simulink model "Copy_of_MMC_test_v3"  (R2020b)
settings: Solver=ode1  StartTime=0.0  StopTime=4  FixedStep=10e-6  RelTol=1e-3
undefined symbols (not defined in the file): DiscIntNeverNeededParam, GRD00_Lg, GRD00_Rg, VSC01_id0
libraries: MMC x12, spsSeriesRLCBranchLib x12, Control_Lib x12, simulink x11, spsThreePhaseSourceLib x5, spsLoadFlowBusLib x4, spsThreePhaseVIMeasurementLib x4, spsThreePhaseBreakerLib x4, spsSecondOrderFilterLib x4, spsThreePhaseParallelRLCLoadLib x3, spsThreePhaseSeriesRLCBranchLib x3, spsCurrentMeasurementLib x2
(part 3 of 3)

== system Copy_of_MMC_test_v3/Mean Model MMC/Control loops/DC part: stored energy control + differential current control/Control Wdiff ==
  Wdiff pu : Inport
  Wdiff_ref pu : Inport  Port=2
  theta : Inport  Port=3
  vv_pu : Inport  Port=4
  Constant : Constant  Value=-2
  Discrete-Time Integrator : DiscreteIntegrator  SampleTime=Time_Step  ICPrevOutput=DiscIntNeverNeededParam  ICPrevScaledInput=DiscIntNeverNeededParam
  Gain5 : Gain  Gain=Vb1/Vdcb
  Gain_i 1 : Gain  Gain=Ki_Wdiff_pu  SaturateOnIntegerOverflow=on  OutDataTypeStr=Inherit: Same as input  ParamDataTypeStr=Inherit: Same as input
  Gain_i 4 : Gain  Gain=Kp_Wdiff_pu  SaturateOnIntegerOverflow=on  OutDataTypeStr=Inherit: Same as input  ParamDataTypeStr=Inherit: Same as input
  Mux1 : Mux  Inputs=3
  Mux2 : Mux  Inputs=3
  Mux3 : Mux  Inputs=3
  Mux5 : Mux  Inputs=2
  Product1 : Product  Inputs=*/*
  Sum2 : Sum  InputSameDT=on  SaturateOnIntegerOverflow=on  OutDataTypeStr=Inherit: Same as first input
  Sum3 : Sum  Inputs=+-  InputSameDT=on  SaturateOnIntegerOverflow=on  OutDataTypeStr=Inherit: Same as first input
  vsa_1 : Fcn  Expr=u(1)*cos(u(4))
  vsa_2 : Fcn  Expr=u(1)-1/2*u(2)-1/2*u(3)
  vsa_3 : Fcn  Expr=u(1)*cos(u(4))+1/3^0.5*u(2)*cos(u(4)+1/2*pi)+1/3^0.5*u(3)*cos(u(4)-1/2*pi)
  vsb_1 : Fcn  Expr=-1/2*u(1)+u(2)-1/2*u(3)
  vsb_2 : Fcn  Expr=u(2)*cos(u(4)-2/3*pi)
  vsb_3 : Fcn  Expr=u(3)*cos(u(4)+2/3*pi)
  vsb_4 : Fcn  Expr=-1/2*u(1)-1/2*u(2)+u(3)
  vsb_5 : Fcn  Expr=1/3^0.5*u(1)*cos(u(4)-7/6*pi)+u(2)*cos(u(4)-2/3*pi)+1/3^0.5*u(3)*cos(u(4)-1/6*pi)
  vsb_6 : Fcn  Expr=1/3^0.5*u(1)*cos(u(4)+7/6*pi)+1/3^0.5*u(2)*cos(u(4)+1/6*pi)+u(3)*cos(u(4)+2/3*pi)
  Idiff ref pu : Outport
  Idiff ref pu1 : Outport  Port=2
  wires:
  Wdiff pu/1 -> Sum3/2
  Wdiff_ref pu/1 -> Sum3/1
  vsb_2/1 -> Mux1/2
  vsa_1/1 -> Mux1/1
  vsb_3/1 -> Mux1/3
  Product1/1 -> Mux5/1  "Idiff_ac_pu"
  vsa_2/1 -> Mux2/1
  vsb_1/1 -> Mux2/2
  vsb_4/1 -> Mux2/3
  vsb_6/1 -> Mux3/3
  vsa_3/1 -> Mux3/1
  vsb_5/1 -> Mux3/2
  Mux5/1 -> vsa_3/1, vsb_5/1, vsb_6/1, vsa_1/1, vsb_2/1, vsb_3/1
  theta/1 -> Mux5/2
  Mux3/1 -> Idiff ref pu/1
  Discrete-Time Integrator/1 -> Sum2/1
  Gain5/1 -> Product1/3
  Gain_i 1/1 -> Discrete-Time Integrator/1
  vv_pu/1 -> Gain5/1
  Sum3/1 -> Gain_i 4/1, Gain_i 1/1
  Sum2/1 -> Product1/1
  Gain_i 4/1 -> Sum2/2
  Mux1/1 -> vsa_2/1, vsb_4/1, vsb_1/1
  Mux2/1 -> Idiff ref pu1/1
  Constant/1 -> Product1/2

== system Copy_of_MMC_test_v3/Mean Model MMC/Control loops/DC part: stored energy control + differential current control/Control Wtot  ==
  note: Reference of i_diff --> adjusting dc power
  note: Energy based control
      |
      | dW
      | ----- = Pdc - Pac --> In this simulation, the energy is regulated by adjusting dc power
      | dt
      |
      | Pdc = PIcontroller*(W_ref - W_mes) + Pac
  note: ac power is considered as a disturbance
  Wtot_pu : Inport
  Wtot ref pu : Inport  Port=2
  p_ac_pu : Inport  Port=3
  Vdc_pu : Inport  Port=4
  Discrete-Time Integrator : DiscreteIntegrator  SampleTime=Time_Step  ICPrevOutput=DiscIntNeverNeededParam  ICPrevScaledInput=DiscIntNeverNeededParam
  Divide1 : Product  Inputs=/*
  Gain1 : Gain  Gain=1/3
  Gain_i 1 : Gain  Gain=Kp_Wtot_pu  SaturateOnIntegerOverflow=on  OutDataTypeStr=Inherit: Same as input  ParamDataTypeStr=Inherit: Same as input
  Gain_i 5 : Gain  Gain=Ki_Wtot_pu  SaturateOnIntegerOverflow=on  OutDataTypeStr=Inherit: Same as input  ParamDataTypeStr=Inherit: Same as input
  Scope{1..4} (4 alike) : Scope
      settings: Tag=op_tm_save_it
  Sum : Sum  Inputs=++|
  Sum1 : Sum  InputSameDT=on  SaturateOnIntegerOverflow=on  OutDataTypeStr=Inherit: Same as first input
  Sum4 : Sum  Inputs=+-  InputSameDT=on  SaturateOnIntegerOverflow=on  OutDataTypeStr=Inherit: Same as first input
  Idiff ref pu : Outport
  wires:
  Sum/1 -> Scope3/1, Divide1/2
  Divide1/1 -> Scope1/1, Idiff ref pu/1  "idiff_ref"
  Vdc_pu/1 -> Divide1/1
  Sum1/1 -> Scope2/1, Sum/2
  Sum4/1 -> Scope4/1, Gain_i 1/1, Gain_i 5/1
  Gain_i 5/1 -> Discrete-Time Integrator/1
  Discrete-Time Integrator/1 -> Sum1/1
  Gain_i 1/1 -> Sum1/2
  Wtot ref pu/1 -> Sum4/1
  Wtot_pu/1 -> Sum4/2
  p_ac_pu/1 -> Gain1/1
  Gain1/1 -> Sum/1

== system Copy_of_MMC_test_v3/Mean Model MMC/Control loops/DC part: stored energy control + differential current control/Differential_current_control ==
  vdc_pu : Inport
  idiff_pu : Inport  Port=2
  idiff_ref_pu : Inport  Port=3
  Discrete-Time Integrator : DiscreteIntegrator  SampleTime=Time_Step  ICPrevOutput=DiscIntNeverNeededParam  ICPrevScaledInput=DiscIntNeverNeededParam
  Gain3 : Gain  Gain=1/2
  Gain_i 1 : Gain  Gain=Diff_CC_kp  SaturateOnIntegerOverflow=on  OutDataTypeStr=Inherit: Same as input  ParamDataTypeStr=Inherit: Same as input
  Gain_i 5 : Gain  Gain=Diff_CC_ki  SaturateOnIntegerOverflow=on  OutDataTypeStr=Inherit: Same as input  ParamDataTypeStr=Inherit: Same as input
  Sum1 : Sum  Inputs=+-  InputSameDT=on  SaturateOnIntegerOverflow=on  OutDataTypeStr=Inherit: Same as first input
  Sum2 : Sum  InputSameDT=on  SaturateOnIntegerOverflow=on  OutDataTypeStr=Inherit: Same as first input
  Sum3 : Sum  Inputs=+-  InputSameDT=on  SaturateOnIntegerOverflow=on  OutDataTypeStr=Inherit: Same as first input
  Vprediff_ref_pu : Outport
  wires:
  idiff_pu/1 -> Sum1/2
  idiff_ref_pu/1 -> Sum1/1
  Sum1/1 -> Gain_i 1/1, Gain_i 5/1
  Gain_i 5/1 -> Discrete-Time Integrator/1
  Gain_i 1/1 -> Sum2/2
  Discrete-Time Integrator/1 -> Sum2/1
  vdc_pu/1 -> Gain3/1
  Gain3/1 -> Sum3/1
  Sum3/1 -> Vprediff_ref_pu/1
  Sum2/1 -> Sum3/2

== system Copy_of_MMC_test_v3/Mean Model MMC/Control loops/DC part: stored energy control + differential current control/Wdiff computation ==
  vctot u_pu : Inport
  vctot l_pu : Inport  Port=2
  Gain10 : Gain  Gain=1/2
  Product : Product
  Product1 : Product
  Second-Order Filter : spsSecondOrderFilterLib/Second-Order Filter  FilterType=Bandstop (Notch)  Fo=fb  Zeta=1  Ts=0  Initialize=on  Vac_Init="[0,  0,  60; 0, 0, 60; 0, 0, 60]"  Vdc_Init=[0, 0, 0]  PlotResponse=off  FreqRange=[0, 500, 1]
      settings: SourceProductBaseCode=PS
  Sum3 : Sum  Inputs=+-
  Wdiff : Outport  PortDimensions=3
  wires:
  vctot u_pu/1 -> Product/2, Product/1
  Sum3/1 -> Gain10/1
  vctot l_pu/1 -> Product1/2, Product1/1
  Product/1 -> Sum3/1
  Product1/1 -> Sum3/2
  Second-Order Filter/1 -> Wdiff/1
  Gain10/1 -> Second-Order Filter/1

== system Copy_of_MMC_test_v3/Mean Model MMC/Control loops/DC part: stored energy control + differential current control/Wtot computation ==
  vctot u_pu : Inport
  vctot l_pu : Inport  Port=2
  Gain10 : Gain  Gain=1/2
  Product : Product
  Product1 : Product
  Second-Order Filter : spsSecondOrderFilterLib/Second-Order Filter  FilterType=Bandstop (Notch)  Fo=2*fb  Zeta=1  Ts=0  Initialize=on  Vac_Init="[0,  0,  60; 0, 0, 60; 0, 0, 60]"  Vdc_Init=[1; 1; 1]  PlotResponse=off  FreqRange=[0, 500, 1]
      settings: SourceProductBaseCode=PS
  Sum3 : Sum
  Wtot : Outport  PortDimensions=3
  wires:
  vctot u_pu/1 -> Product/2, Product/1
  Sum3/1 -> Gain10/1
  vctot l_pu/1 -> Product1/2, Product1/1
  Product/1 -> Sum3/1
  Product1/1 -> Sum3/2
  Second-Order Filter/1 -> Wtot/1
  Gain10/1 -> Second-Order Filter/1

== system Copy_of_MMC_test_v3/Mean Model MMC/Control loops/Power Control Loops1/Inertia Less ==
  P_mes : Inport
  P_set : Inport  Port=2
  delta_PLL : Inport  Port=3
  w_PLL : Inport  Port=4
  Enable : EnablePort
  2*pi : Constant  Value=2*pi
  2*pi1 : Constant
  2*pi2 : Constant  Value=wb*Solver_Time_Step
  2*pi3 : Constant  Value=Val_Freq_Support
  2*pi4 : Constant  Value=0
  Gain : Gain  Gain=Kp_Inertia_Less
  Integrator : Integrator  InitialConditionSource=external
  Integrator2 : Integrator  InitialCondition=(Theta_vsc0)*pi/180-Theta0*pi/180
  Math Function : Math  Operator=mod  SignedPower=on  SaturateOnIntegerOverflow=on
  Sum : Sum  Inputs=|+-
  Sum1 : Sum  Inputs=+++
  Sum2 : Sum  Inputs=|+-
  Sum5 : Sum  Inputs=++|
  Sum6 : Sum  Inputs=|+-
  Sum7 : Sum  Inputs=++|
  Switch : Switch  Criteria=u2 > Threshold  Threshold=0.5
  mp : Gain  Gain=Ki_Inertia_Less
  mp2 : Gain  Gain=1/R
  mp3 : Gain  Gain=wb
  frequency : Outport  VectorParamsAs1DForOutWhenUnconnected=off
  theta : Outport  Port=2  VectorParamsAs1DForOutWhenUnconnected=off
  wires:
  Gain/1 -> Sum/2, Integrator/2
  Integrator/1 -> Sum/1
  2*pi4/1 -> Switch/3
  2*pi3/1 -> Switch/2
  mp2/1 -> Switch/1
  Integrator2/1 -> Sum1/2
  2*pi2/1 -> Sum1/3  "Control Delay Compensation"
  Sum5/1 -> Sum6/2, frequency/1
  w_PLL/1 -> Sum5/2
  delta_PLL/1 -> Sum1/1  "delta_m_ref"
  mp/1 -> Integrator/1
  mp3/1 -> Integrator2/1
  Sum/1 -> Sum5/1, mp3/1  "delta_w"
  Math Function/1 -> theta/1
  Switch/1 -> Sum7/2
  P_mes/1 -> Sum2/2, Gain/1
  Sum7/1 -> Sum2/1  "P_ref"
  P_set/1 -> Sum7/1
  Sum6/1 -> mp2/1
  2*pi1/1 -> Sum6/1
  2*pi/1 -> Math Function/2
  Sum1/1 -> Math Function/1  "delta_m_ref"
  Sum2/1 -> mp/1

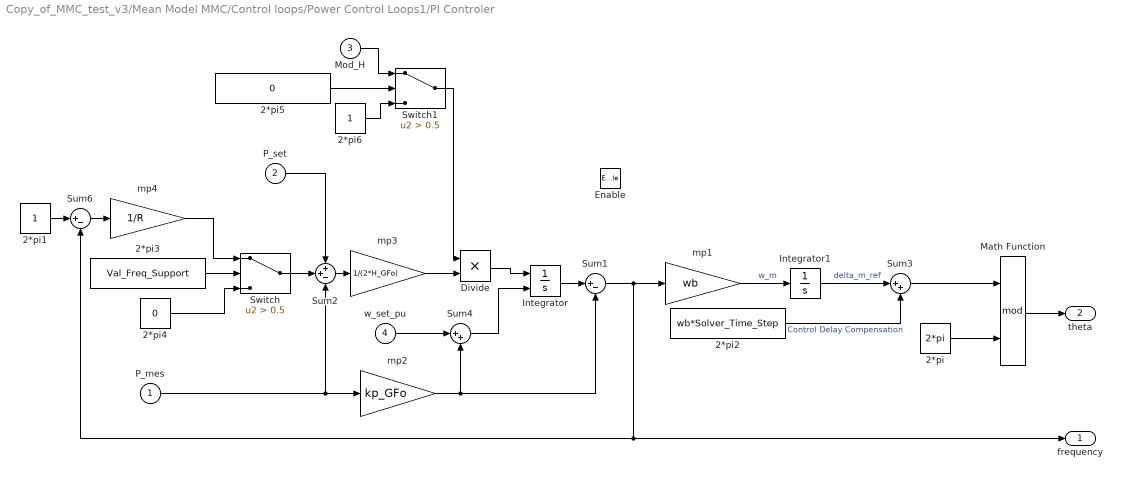
== system Copy_of_MMC_test_v3/Mean Model MMC/Control loops/Power Control Loops1/PI Controler ==
  P_mes : Inport
  P_set : Inport  Port=2
  Mod_H : Inport  Port=3
  w_set_pu : Inport  Port=4
  Enable : EnablePort
  2*pi : Constant  Value=2*pi
  2*pi1 : Constant
  2*pi2 : Constant  Value=wb*Solver_Time_Step
  2*pi3 : Constant  Value=Val_Freq_Support
  2*pi4 : Constant  Value=0
  2*pi5 : Constant  Value=0
  2*pi6 : Constant
  Divide : Product  Inputs=**
  Integrator : Integrator  InitialConditionSource=external
  Integrator1 : Integrator  InitialCondition=(Theta_vsc0)*pi/180
  Math Function : Math  Operator=mod  SignedPower=on  SaturateOnIntegerOverflow=on
  Sum1 : Sum  Inputs=|+-
  Sum2 : Sum  Inputs=++-
  Sum3 : Sum  Inputs=|++
  Sum4 : Sum  Inputs=|++
  Sum6 : Sum  Inputs=|+-
  Switch : Switch  Criteria=u2 > Threshold  Threshold=0.5
  Switch1 : Switch  Criteria=u2 > Threshold  Threshold=0.5
  mp1 : Gain  Gain=wb
  mp2 : Gain  Gain=kp_GFo
  mp3 : Gain  Gain=1/(2*H_GFo)
  mp4 : Gain  Gain=1/R
  frequency : Outport  VectorParamsAs1DForOutWhenUnconnected=off
  theta : Outport  Port=2  VectorParamsAs1DForOutWhenUnconnected=off
  wires:
  Switch1/1 -> Divide/1
  Divide/1 -> Integrator/1
  Mod_H/1 -> Switch1/1
  2*pi6/1 -> Switch1/3
  2*pi5/1 -> Switch1/2
  Switch/1 -> Sum2/2
  2*pi4/1 -> Switch/3
  Sum6/1 -> mp4/1
  2*pi3/1 -> Switch/2
  2*pi1/1 -> Sum6/1
  mp4/1 -> Switch/1
  Sum4/1 -> Integrator/2
  mp3/1 -> Divide/2
  mp2/1 -> Sum4/2, Sum1/2
  P_mes/1 -> mp2/1, Sum2/3
  2*pi2/1 -> Sum3/2  "Control Delay Compensation"
  Sum3/1 -> Math Function/1
  mp1/1 -> Integrator1/1  "w_m"
  Sum1/1 -> Sum6/2, frequency/1, mp1/1
  Integrator/1 -> Sum1/1
  P_set/1 -> Sum2/1
  w_set_pu/1 -> Sum4/1
  2*pi/1 -> Math Function/2
  Math Function/1 -> theta/1
  Integrator1/1 -> Sum3/1  "delta_m_ref"
  Sum2/1 -> mp3/1

== system Copy_of_MMC_test_v3/Mean Model MMC/Control loops/Power Control Loops1/Subsystem ==
  Delta_E_dq : Inport
  Constant : Constant
  Constant1 : Constant  Value=2
  Delay : Delay  DelayLength=1  InitialCondition=1
  Demux : Demux  Outputs=2
  Pow : Math  Operator=pow  SignedPower=on  RndMeth=Zero  SaturateOnIntegerOverflow=on
  Square : Math  Operator=square  SignedPower=on  RndMeth=Zero  SaturateOnIntegerOverflow=on
  Square1 : Math  Operator=square  SignedPower=on  RndMeth=Zero  SaturateOnIntegerOverflow=on
  Sum : Sum  Inputs=|+-
  Sum5 : Sum
  Mod_h : Outport  VectorParamsAs1DForOutWhenUnconnected=off
  wires:
  Delay/1 -> Demux/1
  Sum/1 -> Square/1
  Demux/1 -> Sum/2
  Square1/1 -> Sum5/2
  Sum5/1 -> Pow/1
  Constant/1 -> Sum/1
  Demux/2 -> Square1/1
  Constant1/1 -> Pow/2
  Pow/1 -> Mod_h/1
  Square/1 -> Sum5/1
  Delta_E_dq/1 -> Delay/1

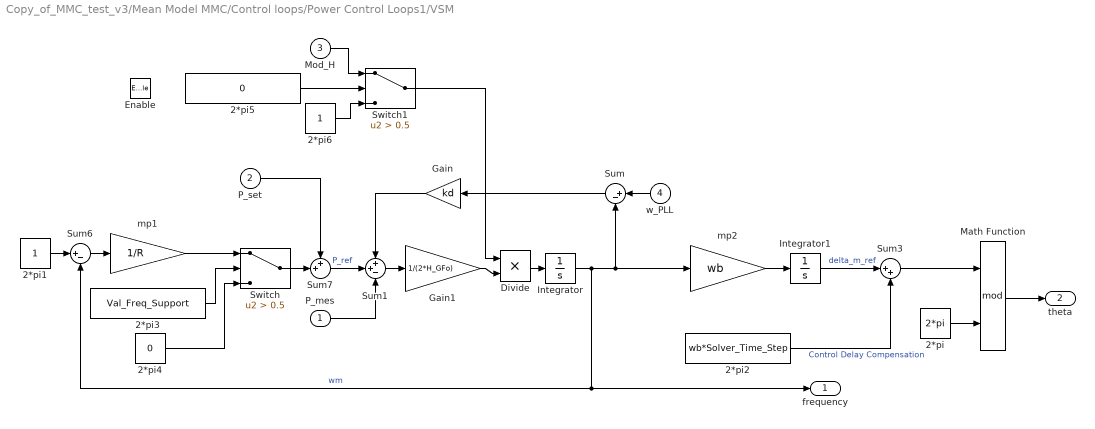
== system Copy_of_MMC_test_v3/Mean Model MMC/Control loops/Power Control Loops1/VSM ==
  P_mes : Inport
  P_set : Inport  Port=2
  Mod_H : Inport  Port=3
  w_PLL : Inport  Port=4
  Enable : EnablePort
  2*pi : Constant  Value=2*pi
  2*pi1 : Constant
  2*pi2 : Constant  Value=wb*Solver_Time_Step
  2*pi3 : Constant  Value=Val_Freq_Support
  2*pi4 : Constant  Value=0
  2*pi5 : Constant  Value=0
  2*pi6 : Constant
  Divide : Product  Inputs=**
  Gain : Gain  Gain=kd
  Gain1 : Gain  Gain=1/(2*H_GFo)
  Integrator : Integrator  InitialCondition=1
  Integrator1 : Integrator  InitialCondition=Theta_vsc0*pi/180
  Math Function : Math  Operator=mod  SignedPower=on  SaturateOnIntegerOverflow=on
  Sum : Sum  Inputs=|+-
  Sum1 : Sum  Inputs=++-
  Sum3 : Sum  Inputs=|++
  Sum6 : Sum  Inputs=|+-
  Sum7 : Sum  Inputs=++|
  Switch : Switch  Criteria=u2 > Threshold  Threshold=0.5
  Switch1 : Switch  Criteria=u2 > Threshold  Threshold=0.5
  mp1 : Gain  Gain=1/R
  mp2 : Gain  Gain=wb
  frequency : Outport  VectorParamsAs1DForOutWhenUnconnected=off
  theta : Outport  Port=2  VectorParamsAs1DForOutWhenUnconnected=off
  wires:
  Switch1/1 -> Divide/1
  Gain1/1 -> Divide/2
  Divide/1 -> Integrator/1
  Mod_H/1 -> Switch1/1
  2*pi6/1 -> Switch1/3
  2*pi5/1 -> Switch1/2
  Sum7/1 -> Sum1/2  "P_ref"
  Sum1/1 -> Gain1/1
  Gain/1 -> Sum1/1
  Sum/1 -> Gain/1
  w_PLL/1 -> Sum/1
  2*pi4/1 -> Switch/3
  2*pi3/1 -> Switch/2
  mp1/1 -> Switch/1
  2*pi1/1 -> Sum6/1
  Sum6/1 -> mp1/1
  P_set/1 -> Sum7/1
  Switch/1 -> Sum7/2
  Sum3/1 -> Math Function/1
  2*pi2/1 -> Sum3/2  "Control Delay Compensation"
  mp2/1 -> Integrator1/1
  P_mes/1 -> Sum1/3
  Integrator/1 -> Sum6/2, frequency/1, mp2/1, Sum/2  "wm"
  Integrator1/1 -> Sum3/1  "delta_m_ref"
  Math Function/1 -> theta/1
  2*pi/1 -> Math Function/2

== system Copy_of_MMC_test_v3/Mean Model MMC/Control loops/Transient Damping Resistance/Filter w_LF ==
  e : Inport
  1/T_LP : Gain  Gain=W_TVR  SaturateOnIntegerOverflow=on  OutDataTypeStr=Inherit: Same as input  ParamDataTypeStr=Inherit: Same as input
  Integrator : Integrator  InitialConditionSource=external  InitialCondition=[VSC01_id0*0.04]
  Sum1 : Sum  Inputs=|+-  InputSameDT=on  SaturateOnIntegerOverflow=on  OutDataTypeStr=Inherit: Same as first input
  s : Outport  VectorParamsAs1DForOutWhenUnconnected=off
  wires:
  e/1 -> Sum1/1, Integrator/2
  Integrator/1 -> s/1, Sum1/2
  1/T_LP/1 -> Integrator/1
  Sum1/1 -> 1/T_LP/1

== system Copy_of_MMC_test_v3/Mean Model MMC/Control loops/VI/dq to phasor ==
  dq_mes : Inport
  Demux : Demux  Outputs=2
      settings: DisplayOption=none
  Sqrt : Sqrt  SaturateOnIntegerOverflow=on
  Sum4 : Sum  Inputs=|++  InputSameDT=on  SaturateOnIntegerOverflow=on  OutDataTypeStr=Inherit: Same as first input
  Vrdird : Product  InputSameDT=on  RndMeth=Zero  SaturateOnIntegerOverflow=on  OutDataTypeStr=Inherit: Same as first input
  Vrqirq : Product  InputSameDT=on  RndMeth=Zero  SaturateOnIntegerOverflow=on  OutDataTypeStr=Inherit: Same as first input
  rms : Outport  VectorParamsAs1DForOutWhenUnconnected=off
  wires:
  Sum4/1 -> Sqrt/1
  Vrqirq/1 -> Sum4/2
  Vrdird/1 -> Sum4/1
  Demux/2 -> Vrqirq/2, Vrqirq/1
  Demux/1 -> Vrdird/2, Vrdird/1
  dq_mes/1 -> Demux/1
  Sqrt/1 -> rms/1

== system Copy_of_MMC_test_v3/Mean Model MMC1/Control loops/Current Limitation/Current control ==
  Ig_dq0* : Inport
  Ig_dq0 : Inport  Port=2
  vg_dq0 : Inport  Port=3
  w : Inport  Port=4
  Demux : Demux  Outputs=2
  Demux1 : Demux  Outputs=2
  Demux2 : Demux  Outputs=2
  Gain Corrector : Gain  Gain=3/(Tr_I_max/1000)*Lt_pu
  Gain Corrector1 : Gain  Gain=3/(Tr_I_max/1000)*Lt_pu
  Mux : Mux  Inputs=2
  Product : Product  RndMeth=Zero
  Product1 : Product  RndMeth=Zero
  Sum : Sum  Inputs=|+-
  Sum2 : Sum  Inputs=|+-
  Sum3 : Sum  Inputs=|++
  Sum5 : Sum  Inputs=++|
  Sum6 : Sum  Inputs=-+|
  Sum7 : Sum  Inputs=++|
  vpcc_abc{1,3..6} (5 alike) : Scope
  w*Lf_pu : Gain  Gain=Lt_pu
  vm : Outport  InitialOutput=0  VectorParamsAs1DForOutWhenUnconnected=off
  wires:
  Demux2/2 -> Sum7/1
  Demux2/1 -> Sum3/2
  w/1 -> vpcc_abc5/1, w*Lf_pu/1
  Sum/1 -> vpcc_abc1/1, Gain Corrector/1
  Sum7/1 -> Mux/2  "Vm_q*"
  Sum3/1 -> Mux/1, vpcc_abc3/1  "Vm_d*"
  Sum5/1 -> Sum7/2
  Product1/1 -> Sum5/1
  Gain Corrector1/1 -> Sum5/2
  Demux/2 -> Sum6/2
  Sum2/1 -> Sum3/1
  Product/1 -> Sum2/2
  Demux1/2 -> Sum6/1, Product/1
  w*Lf_pu/1 -> Product/2, Product1/1
  Gain Corrector/1 -> Sum2/1
  Demux1/1 -> Sum/2, Product1/2
  Demux/1 -> Sum/1
  Ig_dq0/1 -> Demux1/1
  vg_dq0/1 -> Demux2/1, vpcc_abc6/1
  Sum6/1 -> Gain Corrector1/1
  Ig_dq0*/1 -> vpcc_abc4/1, Demux/1
  Mux/1 -> vm/1

== system Copy_of_MMC_test_v3/Mean Model MMC1/Control loops/Current Limitation/Inverse Current control ==
  Vm_dq* : Inport
  Ig_dq : Inport  Port=2
  vg_dq : Inport  Port=3
  w : Inport  Port=4
  Demux : Demux  Outputs=2
  Demux1 : Demux  Outputs=2
  Demux2 : Demux  Outputs=2
  Gain Corrector2 : Gain  Gain=1/(3/(Tr_I_max/1000)*Lt_pu)
  Gain Corrector3 : Gain  Gain=1/(3/(Tr_I_max/1000)*Lt_pu)
  Mux : Mux  Inputs=2
  Product : Product  RndMeth=Zero
  Product1 : Product  RndMeth=Zero
  Sum : Sum  Inputs=|+-
  Sum2 : Sum  Inputs=|++
  Sum3 : Sum  Inputs=|++
  Sum5 : Sum  Inputs=-+|
  Sum6 : Sum  Inputs=-+|
  Sum7 : Sum  Inputs=++|
  w*Lf_pu : Gain  Gain=Lt_pu
  Is_dq* : Outport  InitialOutput=0  VectorParamsAs1DForOutWhenUnconnected=off
  wires:
  vg_dq/1 -> Demux2/1
  Ig_dq/1 -> Demux1/1
  Vm_dq*/1 -> Demux/1
  Demux/1 -> Sum/1
  Demux1/1 -> Sum3/2, Product1/2
  Sum/1 -> Sum2/1
  w*Lf_pu/1 -> Product1/1, Product/2
  Product/1 -> Sum2/2
  Sum2/1 -> Gain Corrector3/1
  Mux/1 -> Is_dq*/1
  Demux/2 -> Sum6/2
  Sum6/1 -> Sum5/2
  Sum5/1 -> Gain Corrector2/1
  Sum3/1 -> Mux/1  "is_d*"
  Sum7/1 -> Mux/2  "is_q*"
  w/1 -> w*Lf_pu/1
  Demux1/2 -> Sum7/1, Product/1
  Gain Corrector3/1 -> Sum3/1
  Demux2/1 -> Sum/2
  Demux2/2 -> Sum6/1
  Product1/1 -> Sum5/1
  Gain Corrector2/1 -> Sum7/2

== system Copy_of_MMC_test_v3/Mean Model MMC1/Control loops/DC part: stored energy control + differential current control/Control Wdiff ==
  Wdiff pu : Inport
  Wdiff_ref pu : Inport  Port=2
  theta : Inport  Port=3
  vv_pu : Inport  Port=4
  Constant : Constant  Value=-2
  Discrete-Time Integrator : DiscreteIntegrator  SampleTime=Time_Step  ICPrevOutput=DiscIntNeverNeededParam  ICPrevScaledInput=DiscIntNeverNeededParam
  Gain5 : Gain  Gain=Vb1/Vdcb
  Gain_i 1 : Gain  Gain=Ki_Wdiff_pu  SaturateOnIntegerOverflow=on  OutDataTypeStr=Inherit: Same as input  ParamDataTypeStr=Inherit: Same as input
  Gain_i 4 : Gain  Gain=Kp_Wdiff_pu  SaturateOnIntegerOverflow=on  OutDataTypeStr=Inherit: Same as input  ParamDataTypeStr=Inherit: Same as input
  Mux1 : Mux  Inputs=3
  Mux2 : Mux  Inputs=3
  Mux3 : Mux  Inputs=3
  Mux5 : Mux  Inputs=2
  Product1 : Product  Inputs=*/*
  Sum2 : Sum  InputSameDT=on  SaturateOnIntegerOverflow=on  OutDataTypeStr=Inherit: Same as first input
  Sum3 : Sum  Inputs=+-  InputSameDT=on  SaturateOnIntegerOverflow=on  OutDataTypeStr=Inherit: Same as first input
  vsa_1 : Fcn  Expr=u(1)*cos(u(4))
  vsa_2 : Fcn  Expr=u(1)-1/2*u(2)-1/2*u(3)
  vsa_3 : Fcn  Expr=u(1)*cos(u(4))+1/3^0.5*u(2)*cos(u(4)+1/2*pi)+1/3^0.5*u(3)*cos(u(4)-1/2*pi)
  vsb_1 : Fcn  Expr=-1/2*u(1)+u(2)-1/2*u(3)
  vsb_2 : Fcn  Expr=u(2)*cos(u(4)-2/3*pi)
  vsb_3 : Fcn  Expr=u(3)*cos(u(4)+2/3*pi)
  vsb_4 : Fcn  Expr=-1/2*u(1)-1/2*u(2)+u(3)
  vsb_5 : Fcn  Expr=1/3^0.5*u(1)*cos(u(4)-7/6*pi)+u(2)*cos(u(4)-2/3*pi)+1/3^0.5*u(3)*cos(u(4)-1/6*pi)
  vsb_6 : Fcn  Expr=1/3^0.5*u(1)*cos(u(4)+7/6*pi)+1/3^0.5*u(2)*cos(u(4)+1/6*pi)+u(3)*cos(u(4)+2/3*pi)
  Idiff ref pu : Outport
  Idiff ref pu1 : Outport  Port=2
  wires:
  Wdiff pu/1 -> Sum3/2
  Wdiff_ref pu/1 -> Sum3/1
  vsb_2/1 -> Mux1/2
  vsa_1/1 -> Mux1/1
  vsb_3/1 -> Mux1/3
  Product1/1 -> Mux5/1  "Idiff_ac_pu"
  vsa_2/1 -> Mux2/1
  vsb_1/1 -> Mux2/2
  vsb_4/1 -> Mux2/3
  vsb_6/1 -> Mux3/3
  vsa_3/1 -> Mux3/1
  vsb_5/1 -> Mux3/2
  Mux5/1 -> vsa_3/1, vsb_5/1, vsb_6/1, vsa_1/1, vsb_2/1, vsb_3/1
  theta/1 -> Mux5/2
  Mux3/1 -> Idiff ref pu/1
  Discrete-Time Integrator/1 -> Sum2/1
  Gain5/1 -> Product1/3
  Gain_i 1/1 -> Discrete-Time Integrator/1
  vv_pu/1 -> Gain5/1
  Sum3/1 -> Gain_i 4/1, Gain_i 1/1
  Sum2/1 -> Product1/1
  Gain_i 4/1 -> Sum2/2
  Mux1/1 -> vsa_2/1, vsb_4/1, vsb_1/1
  Mux2/1 -> Idiff ref pu1/1
  Constant/1 -> Product1/2

== system Copy_of_MMC_test_v3/Mean Model MMC1/Control loops/DC part: stored energy control + differential current control/Control Wtot  ==
  note: Reference of i_diff --> adjusting dc power
  note: Energy based control
      |
      | dW
      | ----- = Pdc - Pac --> In this simulation, the energy is regulated by adjusting dc power
      | dt
      |
      | Pdc = PIcontroller*(W_ref - W_mes) + Pac
  note: ac power is considered as a disturbance
  Wtot_pu : Inport
  Wtot ref pu : Inport  Port=2
  p_ac_pu : Inport  Port=3
  Vdc_pu : Inport  Port=4
  Discrete-Time Integrator : DiscreteIntegrator  SampleTime=Time_Step  ICPrevOutput=DiscIntNeverNeededParam  ICPrevScaledInput=DiscIntNeverNeededParam
  Divide1 : Product  Inputs=/*
  Gain1 : Gain  Gain=1/3
  Gain_i 1 : Gain  Gain=Kp_Wtot_pu  SaturateOnIntegerOverflow=on  OutDataTypeStr=Inherit: Same as input  ParamDataTypeStr=Inherit: Same as input
  Gain_i 5 : Gain  Gain=Ki_Wtot_pu  SaturateOnIntegerOverflow=on  OutDataTypeStr=Inherit: Same as input  ParamDataTypeStr=Inherit: Same as input
  Scope{1..4} (4 alike) : Scope
      settings: Tag=op_tm_save_it
  Sum : Sum  Inputs=++|
  Sum1 : Sum  InputSameDT=on  SaturateOnIntegerOverflow=on  OutDataTypeStr=Inherit: Same as first input
  Sum4 : Sum  Inputs=+-  InputSameDT=on  SaturateOnIntegerOverflow=on  OutDataTypeStr=Inherit: Same as first input
  Idiff ref pu : Outport
  wires:
  Sum/1 -> Scope3/1, Divide1/2
  Divide1/1 -> Scope1/1, Idiff ref pu/1  "idiff_ref"
  Vdc_pu/1 -> Divide1/1
  Sum1/1 -> Scope2/1, Sum/2
  Sum4/1 -> Scope4/1, Gain_i 1/1, Gain_i 5/1
  Gain_i 5/1 -> Discrete-Time Integrator/1
  Discrete-Time Integrator/1 -> Sum1/1
  Gain_i 1/1 -> Sum1/2
  Wtot ref pu/1 -> Sum4/1
  Wtot_pu/1 -> Sum4/2
  p_ac_pu/1 -> Gain1/1
  Gain1/1 -> Sum/1

== system Copy_of_MMC_test_v3/Mean Model MMC1/Control loops/DC part: stored energy control + differential current control/Differential_current_control ==
  vdc_pu : Inport
  idiff_pu : Inport  Port=2
  idiff_ref_pu : Inport  Port=3
  Discrete-Time Integrator : DiscreteIntegrator  SampleTime=Time_Step  ICPrevOutput=DiscIntNeverNeededParam  ICPrevScaledInput=DiscIntNeverNeededParam
  Gain3 : Gain  Gain=1/2
  Gain_i 1 : Gain  Gain=Diff_CC_kp  SaturateOnIntegerOverflow=on  OutDataTypeStr=Inherit: Same as input  ParamDataTypeStr=Inherit: Same as input
  Gain_i 5 : Gain  Gain=Diff_CC_ki  SaturateOnIntegerOverflow=on  OutDataTypeStr=Inherit: Same as input  ParamDataTypeStr=Inherit: Same as input
  Sum1 : Sum  Inputs=+-  InputSameDT=on  SaturateOnIntegerOverflow=on  OutDataTypeStr=Inherit: Same as first input
  Sum2 : Sum  InputSameDT=on  SaturateOnIntegerOverflow=on  OutDataTypeStr=Inherit: Same as first input
  Sum3 : Sum  Inputs=+-  InputSameDT=on  SaturateOnIntegerOverflow=on  OutDataTypeStr=Inherit: Same as first input
  Vprediff_ref_pu : Outport
  wires:
  idiff_pu/1 -> Sum1/2
  idiff_ref_pu/1 -> Sum1/1
  Sum1/1 -> Gain_i 1/1, Gain_i 5/1
  Gain_i 5/1 -> Discrete-Time Integrator/1
  Gain_i 1/1 -> Sum2/2
  Discrete-Time Integrator/1 -> Sum2/1
  vdc_pu/1 -> Gain3/1
  Gain3/1 -> Sum3/1
  Sum3/1 -> Vprediff_ref_pu/1
  Sum2/1 -> Sum3/2

== system Copy_of_MMC_test_v3/Mean Model MMC1/Control loops/DC part: stored energy control + differential current control/Wdiff computation ==
  vctot u_pu : Inport
  vctot l_pu : Inport  Port=2
  Gain10 : Gain  Gain=1/2
  Product : Product
  Product1 : Product
  Second-Order Filter : spsSecondOrderFilterLib/Second-Order Filter  FilterType=Bandstop (Notch)  Fo=fb  Zeta=1  Ts=0  Initialize=on  Vac_Init="[0,  0,  60; 0, 0, 60; 0, 0, 60]"  Vdc_Init=[0, 0, 0]  PlotResponse=off  FreqRange=[0, 500, 1]
      settings: SourceProductBaseCode=PS
  Sum3 : Sum  Inputs=+-
  Wdiff : Outport  PortDimensions=3
  wires:
  vctot u_pu/1 -> Product/2, Product/1
  Sum3/1 -> Gain10/1
  vctot l_pu/1 -> Product1/2, Product1/1
  Product/1 -> Sum3/1
  Product1/1 -> Sum3/2
  Second-Order Filter/1 -> Wdiff/1
  Gain10/1 -> Second-Order Filter/1

== system Copy_of_MMC_test_v3/Mean Model MMC1/Control loops/DC part: stored energy control + differential current control/Wtot computation ==
  vctot u_pu : Inport
  vctot l_pu : Inport  Port=2
  Gain10 : Gain  Gain=1/2
  Product : Product
  Product1 : Product
  Second-Order Filter : spsSecondOrderFilterLib/Second-Order Filter  FilterType=Bandstop (Notch)  Fo=2*fb  Zeta=1  Ts=0  Initialize=on  Vac_Init="[0,  0,  60; 0, 0, 60; 0, 0, 60]"  Vdc_Init=[1; 1; 1]  PlotResponse=off  FreqRange=[0, 500, 1]
      settings: SourceProductBaseCode=PS
  Sum3 : Sum
  Wtot : Outport  PortDimensions=3
  wires:
  vctot u_pu/1 -> Product/2, Product/1
  Sum3/1 -> Gain10/1
  vctot l_pu/1 -> Product1/2, Product1/1
  Product/1 -> Sum3/1
  Product1/1 -> Sum3/2
  Second-Order Filter/1 -> Wtot/1
  Gain10/1 -> Second-Order Filter/1

== system Copy_of_MMC_test_v3/Mean Model MMC1/Control loops/Power Control Loops/Inertia Less ==
  P_mes : Inport
  P_set : Inport  Port=2
  delta_PLL : Inport  Port=3
  w_PLL : Inport  Port=4
  Enable : EnablePort
  2*pi : Constant  Value=2*pi
  2*pi1 : Constant
  2*pi2 : Constant  Value=wb*Solver_Time_Step
  2*pi3 : Constant  Value=Val_Freq_Support
  2*pi4 : Constant  Value=0
  Gain : Gain  Gain=Kp_Inertia_Less
  Integrator : Integrator  InitialConditionSource=external
  Integrator2 : Integrator  InitialCondition=(Theta_vsc0)*pi/180-Theta0*pi/180
  Math Function : Math  Operator=mod  SignedPower=on  SaturateOnIntegerOverflow=on
  Sum : Sum  Inputs=|+-
  Sum1 : Sum  Inputs=+++
  Sum2 : Sum  Inputs=|+-
  Sum5 : Sum  Inputs=++|
  Sum6 : Sum  Inputs=|+-
  Sum7 : Sum  Inputs=++|
  Switch : Switch  Criteria=u2 > Threshold  Threshold=0.5
  mp : Gain  Gain=Ki_Inertia_Less
  mp2 : Gain  Gain=1/R
  mp3 : Gain  Gain=wb
  frequency : Outport  VectorParamsAs1DForOutWhenUnconnected=off
  theta : Outport  Port=2  VectorParamsAs1DForOutWhenUnconnected=off
  wires:
  Gain/1 -> Sum/2, Integrator/2
  Integrator/1 -> Sum/1
  2*pi4/1 -> Switch/3
  2*pi3/1 -> Switch/2
  mp2/1 -> Switch/1
  Integrator2/1 -> Sum1/2
  2*pi2/1 -> Sum1/3  "Control Delay Compensation"
  Sum5/1 -> Sum6/2, frequency/1
  w_PLL/1 -> Sum5/2
  delta_PLL/1 -> Sum1/1  "delta_m_ref"
  mp/1 -> Integrator/1
  mp3/1 -> Integrator2/1
  Sum/1 -> Sum5/1, mp3/1  "delta_w"
  Math Function/1 -> theta/1
  Switch/1 -> Sum7/2
  P_mes/1 -> Sum2/2, Gain/1
  Sum7/1 -> Sum2/1  "P_ref"
  P_set/1 -> Sum7/1
  Sum6/1 -> mp2/1
  2*pi1/1 -> Sum6/1
  2*pi/1 -> Math Function/2
  Sum1/1 -> Math Function/1  "delta_m_ref"
  Sum2/1 -> mp/1

== system Copy_of_MMC_test_v3/Mean Model MMC1/Control loops/Power Control Loops/PI Controler ==
  P_mes : Inport
  P_set : Inport  Port=2
  w_set_pu : Inport  Port=3
  Enable : EnablePort
  2*pi : Constant  Value=2*pi
  2*pi1 : Constant
  2*pi2 : Constant  Value=wb*Solver_Time_Step
  2*pi3 : Constant  Value=Val_Freq_Support
  2*pi4 : Constant  Value=0
  Integrator : Integrator  InitialConditionSource=external
  Integrator1 : Integrator  InitialCondition=(Theta_vsc0)*pi/180
  Math Function : Math  Operator=mod  SignedPower=on  SaturateOnIntegerOverflow=on
  Sum1 : Sum  Inputs=|+-
  Sum2 : Sum  Inputs=++-
  Sum3 : Sum  Inputs=|++
  Sum4 : Sum  Inputs=|++
  Sum6 : Sum  Inputs=|+-
  Switch : Switch  Criteria=u2 > Threshold  Threshold=0.5
  mp1 : Gain  Gain=wb
  mp2 : Gain  Gain=kp_GFo
  mp3 : Gain  Gain=1/(2*H_GFo)
  mp4 : Gain  Gain=1/R
  frequency : Outport  VectorParamsAs1DForOutWhenUnconnected=off
  theta : Outport  Port=2  VectorParamsAs1DForOutWhenUnconnected=off
  wires:
  Switch/1 -> Sum2/2
  2*pi4/1 -> Switch/3
  Sum6/1 -> mp4/1
  2*pi3/1 -> Switch/2
  2*pi1/1 -> Sum6/1
  mp4/1 -> Switch/1
  Sum4/1 -> Integrator/2
  mp3/1 -> Integrator/1
  mp2/1 -> Sum4/2, Sum1/2
  P_mes/1 -> mp2/1, Sum2/3
  2*pi2/1 -> Sum3/2  "Control Delay Compensation"
  Sum3/1 -> Math Function/1
  mp1/1 -> Integrator1/1  "w_m"
  Sum1/1 -> Sum6/2, frequency/1, mp1/1
  Integrator/1 -> Sum1/1
  P_set/1 -> Sum2/1
  w_set_pu/1 -> Sum4/1
  2*pi/1 -> Math Function/2
  Math Function/1 -> theta/1
  Integrator1/1 -> Sum3/1  "delta_m_ref"
  Sum2/1 -> mp3/1

== system Copy_of_MMC_test_v3/Mean Model MMC1/Control loops/Power Control Loops/VSM ==
  P_mes : Inport
  P_set : Inport  Port=2
  w_PLL : Inport  Port=3
  Enable : EnablePort
  2*pi : Constant  Value=2*pi
  2*pi1 : Constant
  2*pi2 : Constant  Value=wb*Solver_Time_Step
  2*pi3 : Constant  Value=Val_Freq_Support
  2*pi4 : Constant  Value=0
  Gain : Gain  Gain=kd
  Gain1 : Gain  Gain=1/(2*H_GFo)
  Integrator : Integrator  InitialCondition=1
  Integrator1 : Integrator  InitialCondition=Theta_vsc0*pi/180
  Math Function : Math  Operator=mod  SignedPower=on  SaturateOnIntegerOverflow=on
  Sum : Sum  Inputs=|+-
  Sum1 : Sum  Inputs=++-
  Sum3 : Sum  Inputs=|++
  Sum6 : Sum  Inputs=|+-
  Sum7 : Sum  Inputs=++|
  Switch : Switch  Criteria=u2 > Threshold  Threshold=0.5
  mp1 : Gain  Gain=1/R
  mp2 : Gain  Gain=wb
  frequency : Outport  VectorParamsAs1DForOutWhenUnconnected=off
  theta : Outport  Port=2  VectorParamsAs1DForOutWhenUnconnected=off
  wires:
  Gain1/1 -> Integrator/1
  Sum7/1 -> Sum1/2  "P_ref"
  Sum1/1 -> Gain1/1
  Gain/1 -> Sum1/1
  Sum/1 -> Gain/1
  w_PLL/1 -> Sum/1
  2*pi4/1 -> Switch/3
  2*pi3/1 -> Switch/2
  mp1/1 -> Switch/1
  2*pi1/1 -> Sum6/1
  Sum6/1 -> mp1/1
  P_set/1 -> Sum7/1
  Switch/1 -> Sum7/2
  Sum3/1 -> Math Function/1
  2*pi2/1 -> Sum3/2  "Control Delay Compensation"
  mp2/1 -> Integrator1/1
  P_mes/1 -> Sum1/3
  Integrator/1 -> Sum6/2, frequency/1, mp2/1, Sum/2  "wm"
  Integrator1/1 -> Sum3/1  "delta_m_ref"
  Math Function/1 -> theta/1
  2*pi/1 -> Math Function/2

== system Copy_of_MMC_test_v3/Mean Model MMC1/Control loops/Power Control Loops1/Inertia Less ==
  P_mes : Inport
  P_set : Inport  Port=2
  delta_PLL : Inport  Port=3
  w_PLL : Inport  Port=4
  Enable : EnablePort
  2*pi : Constant  Value=2*pi
  2*pi1 : Constant
  2*pi2 : Constant  Value=wb*Solver_Time_Step
  2*pi3 : Constant  Value=Val_Freq_Support
  2*pi4 : Constant  Value=0
  Gain : Gain  Gain=Kp_Inertia_Less
  Integrator : Integrator  InitialConditionSource=external
  Integrator2 : Integrator  InitialCondition=(Theta_vsc0)*pi/180-Theta0*pi/180
  Math Function : Math  Operator=mod  SignedPower=on  SaturateOnIntegerOverflow=on
  Sum : Sum  Inputs=|+-
  Sum1 : Sum  Inputs=+++
  Sum2 : Sum  Inputs=|+-
  Sum5 : Sum  Inputs=++|
  Sum6 : Sum  Inputs=|+-
  Sum7 : Sum  Inputs=++|
  Switch : Switch  Criteria=u2 > Threshold  Threshold=0.5
  mp : Gain  Gain=Ki_Inertia_Less
  mp2 : Gain  Gain=1/R
  mp3 : Gain  Gain=wb
  frequency : Outport  VectorParamsAs1DForOutWhenUnconnected=off
  theta : Outport  Port=2  VectorParamsAs1DForOutWhenUnconnected=off
  wires:
  Gain/1 -> Sum/2, Integrator/2
  Integrator/1 -> Sum/1
  2*pi4/1 -> Switch/3
  2*pi3/1 -> Switch/2
  mp2/1 -> Switch/1
  Integrator2/1 -> Sum1/2
  2*pi2/1 -> Sum1/3  "Control Delay Compensation"
  Sum5/1 -> Sum6/2, frequency/1
  w_PLL/1 -> Sum5/2
  delta_PLL/1 -> Sum1/1  "delta_m_ref"
  mp/1 -> Integrator/1
  mp3/1 -> Integrator2/1
  Sum/1 -> Sum5/1, mp3/1  "delta_w"
  Math Function/1 -> theta/1
  Switch/1 -> Sum7/2
  P_mes/1 -> Sum2/2, Gain/1
  Sum7/1 -> Sum2/1  "P_ref"
  P_set/1 -> Sum7/1
  Sum6/1 -> mp2/1
  2*pi1/1 -> Sum6/1
  2*pi/1 -> Math Function/2
  Sum1/1 -> Math Function/1  "delta_m_ref"
  Sum2/1 -> mp/1

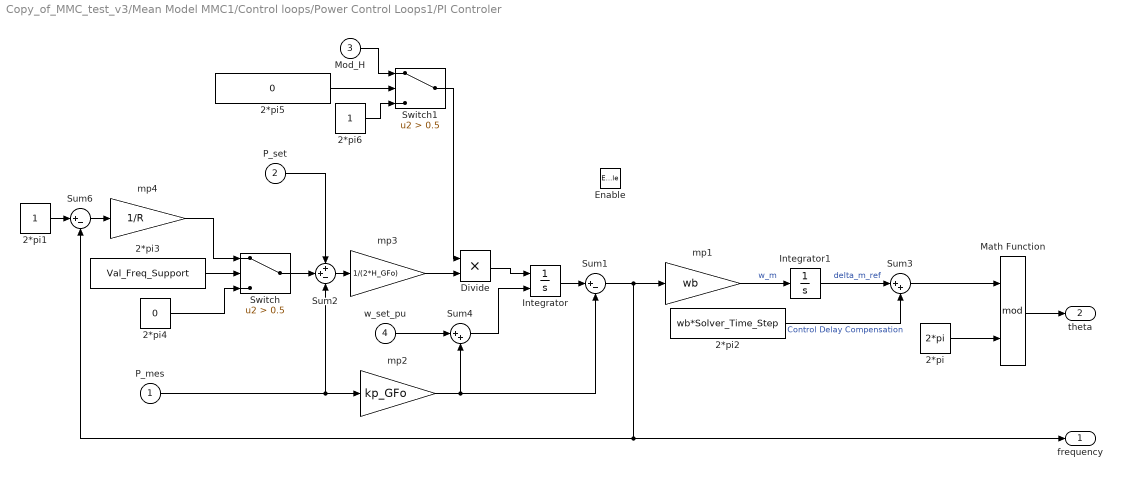
== system Copy_of_MMC_test_v3/Mean Model MMC1/Control loops/Power Control Loops1/PI Controler ==
  P_mes : Inport
  P_set : Inport  Port=2
  Mod_H : Inport  Port=3
  w_set_pu : Inport  Port=4
  Enable : EnablePort
  2*pi : Constant  Value=2*pi
  2*pi1 : Constant
  2*pi2 : Constant  Value=wb*Solver_Time_Step
  2*pi3 : Constant  Value=Val_Freq_Support
  2*pi4 : Constant  Value=0
  2*pi5 : Constant  Value=0
  2*pi6 : Constant
  Divide : Product  Inputs=**
  Integrator : Integrator  InitialConditionSource=external
  Integrator1 : Integrator  InitialCondition=(Theta_vsc0)*pi/180
  Math Function : Math  Operator=mod  SignedPower=on  SaturateOnIntegerOverflow=on
  Sum1 : Sum  Inputs=|+-
  Sum2 : Sum  Inputs=++-
  Sum3 : Sum  Inputs=|++
  Sum4 : Sum  Inputs=|++
  Sum6 : Sum  Inputs=|+-
  Switch : Switch  Criteria=u2 > Threshold  Threshold=0.5
  Switch1 : Switch  Criteria=u2 > Threshold  Threshold=0.5
  mp1 : Gain  Gain=wb
  mp2 : Gain  Gain=kp_GFo
  mp3 : Gain  Gain=1/(2*H_GFo)
  mp4 : Gain  Gain=1/R
  frequency : Outport  VectorParamsAs1DForOutWhenUnconnected=off
  theta : Outport  Port=2  VectorParamsAs1DForOutWhenUnconnected=off
  wires:
  Switch1/1 -> Divide/1
  Divide/1 -> Integrator/1
  Mod_H/1 -> Switch1/1
  2*pi6/1 -> Switch1/3
  2*pi5/1 -> Switch1/2
  Switch/1 -> Sum2/2
  2*pi4/1 -> Switch/3
  Sum6/1 -> mp4/1
  2*pi3/1 -> Switch/2
  2*pi1/1 -> Sum6/1
  mp4/1 -> Switch/1
  Sum4/1 -> Integrator/2
  mp3/1 -> Divide/2
  mp2/1 -> Sum4/2, Sum1/2
  P_mes/1 -> mp2/1, Sum2/3
  2*pi2/1 -> Sum3/2  "Control Delay Compensation"
  Sum3/1 -> Math Function/1
  mp1/1 -> Integrator1/1  "w_m"
  Sum1/1 -> Sum6/2, frequency/1, mp1/1
  Integrator/1 -> Sum1/1
  P_set/1 -> Sum2/1
  w_set_pu/1 -> Sum4/1
  2*pi/1 -> Math Function/2
  Math Function/1 -> theta/1
  Integrator1/1 -> Sum3/1  "delta_m_ref"
  Sum2/1 -> mp3/1

== system Copy_of_MMC_test_v3/Mean Model MMC1/Control loops/Power Control Loops1/Subsystem ==
  Delta_E_dq : Inport
  Constant : Constant
  Constant1 : Constant  Value=2
  Delay : Delay  DelayLength=1  InitialCondition=1
  Demux : Demux  Outputs=2
  Pow : Math  Operator=pow  SignedPower=on  RndMeth=Zero  SaturateOnIntegerOverflow=on
  Square : Math  Operator=square  SignedPower=on  RndMeth=Zero  SaturateOnIntegerOverflow=on
  Square1 : Math  Operator=square  SignedPower=on  RndMeth=Zero  SaturateOnIntegerOverflow=on
  Sum : Sum  Inputs=|+-
  Sum5 : Sum
  Mod_h : Outport  VectorParamsAs1DForOutWhenUnconnected=off
  wires:
  Delay/1 -> Demux/1
  Sum/1 -> Square/1
  Demux/1 -> Sum/2
  Square1/1 -> Sum5/2
  Sum5/1 -> Pow/1
  Constant/1 -> Sum/1
  Demux/2 -> Square1/1
  Constant1/1 -> Pow/2
  Pow/1 -> Mod_h/1
  Square/1 -> Sum5/1
  Delta_E_dq/1 -> Delay/1

== system Copy_of_MMC_test_v3/Mean Model MMC1/Control loops/Power Control Loops1/VSM ==
  P_mes : Inport
  P_set : Inport  Port=2
  Mod_H : Inport  Port=3
  w_PLL : Inport  Port=4
  Enable : EnablePort
  2*pi : Constant  Value=2*pi
  2*pi1 : Constant
  2*pi2 : Constant  Value=wb*Solver_Time_Step
  2*pi3 : Constant  Value=Val_Freq_Support
  2*pi4 : Constant  Value=0
  2*pi5 : Constant  Value=0
  2*pi6 : Constant
  Divide : Product  Inputs=**
  Gain : Gain  Gain=kd
  Gain1 : Gain  Gain=1/(2*H_GFo)
  Integrator : Integrator  InitialCondition=1
  Integrator1 : Integrator  InitialCondition=Theta_vsc0*pi/180
  Math Function : Math  Operator=mod  SignedPower=on  SaturateOnIntegerOverflow=on
  Sum : Sum  Inputs=|+-
  Sum1 : Sum  Inputs=++-
  Sum3 : Sum  Inputs=|++
  Sum6 : Sum  Inputs=|+-
  Sum7 : Sum  Inputs=++|
  Switch : Switch  Criteria=u2 > Threshold  Threshold=0.5
  Switch1 : Switch  Criteria=u2 > Threshold  Threshold=0.5
  mp1 : Gain  Gain=1/R
  mp2 : Gain  Gain=wb
  frequency : Outport  VectorParamsAs1DForOutWhenUnconnected=off
  theta : Outport  Port=2  VectorParamsAs1DForOutWhenUnconnected=off
  wires:
  Switch1/1 -> Divide/1
  Gain1/1 -> Divide/2
  Divide/1 -> Integrator/1
  Mod_H/1 -> Switch1/1
  2*pi6/1 -> Switch1/3
  2*pi5/1 -> Switch1/2
  Sum7/1 -> Sum1/2  "P_ref"
  Sum1/1 -> Gain1/1
  Gain/1 -> Sum1/1
  Sum/1 -> Gain/1
  w_PLL/1 -> Sum/1
  2*pi4/1 -> Switch/3
  2*pi3/1 -> Switch/2
  mp1/1 -> Switch/1
  2*pi1/1 -> Sum6/1
  Sum6/1 -> mp1/1
  P_set/1 -> Sum7/1
  Switch/1 -> Sum7/2
  Sum3/1 -> Math Function/1
  2*pi2/1 -> Sum3/2  "Control Delay Compensation"
  mp2/1 -> Integrator1/1
  P_mes/1 -> Sum1/3
  Integrator/1 -> Sum6/2, frequency/1, mp2/1, Sum/2  "wm"
  Integrator1/1 -> Sum3/1  "delta_m_ref"
  Math Function/1 -> theta/1
  2*pi/1 -> Math Function/2

== system Copy_of_MMC_test_v3/Mean Model MMC1/Control loops/Transient Damping Resistance/Filter w_LF ==
  e : Inport
  1/T_LP : Gain  Gain=W_TVR  SaturateOnIntegerOverflow=on  OutDataTypeStr=Inherit: Same as input  ParamDataTypeStr=Inherit: Same as input
  Integrator : Integrator  InitialConditionSource=external  InitialCondition=[VSC01_id0*0.04]
  Sum1 : Sum  Inputs=|+-  InputSameDT=on  SaturateOnIntegerOverflow=on  OutDataTypeStr=Inherit: Same as first input
  s : Outport  VectorParamsAs1DForOutWhenUnconnected=off
  wires:
  e/1 -> Sum1/1, Integrator/2
  Integrator/1 -> s/1, Sum1/2
  1/T_LP/1 -> Integrator/1
  Sum1/1 -> 1/T_LP/1

== system Copy_of_MMC_test_v3/Mean Model MMC1/Control loops/VI/dq to phasor ==
  dq_mes : Inport
  Demux : Demux  Outputs=2
      settings: DisplayOption=none
  Sqrt : Sqrt  SaturateOnIntegerOverflow=on
  Sum4 : Sum  Inputs=|++  InputSameDT=on  SaturateOnIntegerOverflow=on  OutDataTypeStr=Inherit: Same as first input
  Vrdird : Product  InputSameDT=on  RndMeth=Zero  SaturateOnIntegerOverflow=on  OutDataTypeStr=Inherit: Same as first input
  Vrqirq : Product  InputSameDT=on  RndMeth=Zero  SaturateOnIntegerOverflow=on  OutDataTypeStr=Inherit: Same as first input
  rms : Outport  VectorParamsAs1DForOutWhenUnconnected=off
  wires:
  Sum4/1 -> Sqrt/1
  Vrqirq/1 -> Sum4/2
  Vrdird/1 -> Sum4/1
  Demux/2 -> Vrqirq/2, Vrqirq/1
  Demux/1 -> Vrdird/2, Vrdird/1
  dq_mes/1 -> Demux/1
  Sqrt/1 -> rms/1
